simulink model "OnlineEstimation_MIL"  (R2024a)
settings: Solver=FixedStepAuto  StartTime=0.0  StopTime=50  FixedStep=0.001  RelTol=1e-3
undefined symbols (not defined in the file or in its folder): magnitude
libraries: fl_lib x16, nesl_utility x10, simulink x4, ee_lib x4, fl_ps_legacy_lib x2, ctrlSharedLib x2, eeGeneralControl x2, sdl_lib x1
settings Model: Creator=rocke  LastModifiedBy=rocke

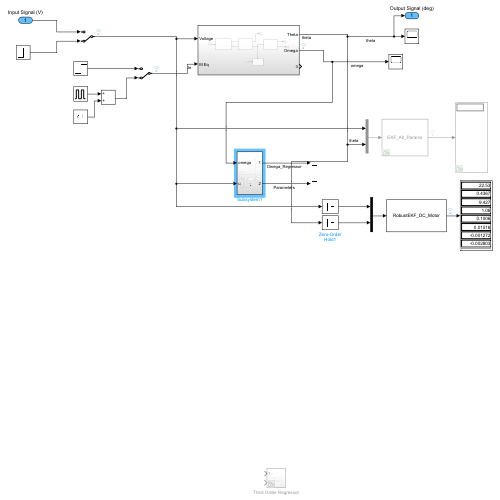
[thumbnail: Simulink's stored preview of the top-level diagram]
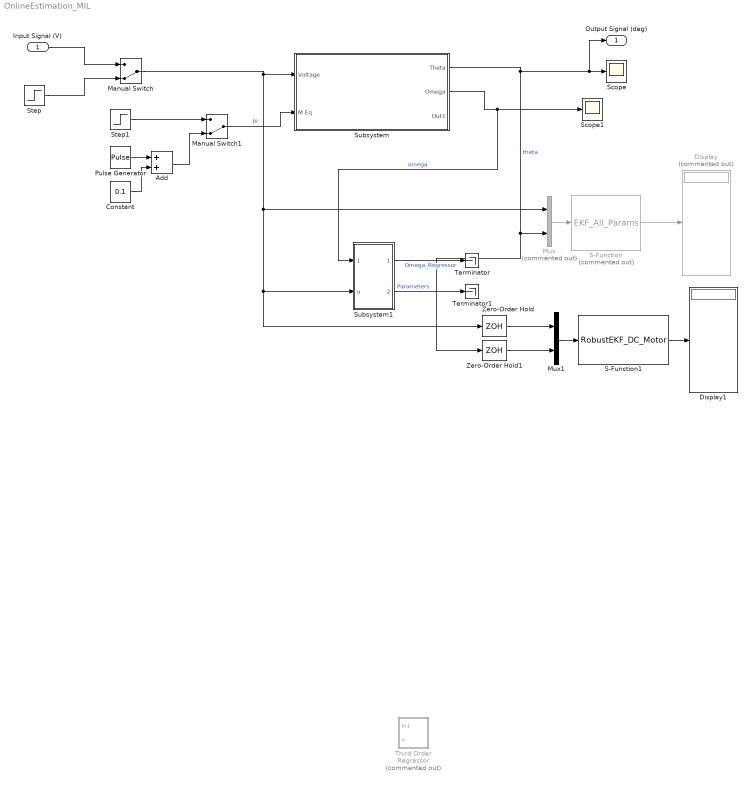
== system OnlineEstimation_MIL ==
  Input Signal (V) : Inport
  Add : Sum
  Constant : Constant  Value=0.1
  Display : Display  Commented=on
  Display1 : Display
  Manual Switch : ManualSwitch  CurrentSetting=0
  Manual Switch1 : ManualSwitch  CurrentSetting=0
  Mux : Mux  Commented=on  Inputs=2
  Mux1 : Mux  Inputs=2
  Pulse Generator : DiscretePulseGenerator  PulseType=Time based  Amplitude=0.2  Period=10  PulseWidth=50  PhaseDelay=5
  S-Function : S-Function  Commented=on  FunctionName=EKF_All_Params  SFunctionDeploymentMode=off  EnableBusSupport=off
  S-Function1 : S-Function  FunctionName=RobustEKF_DC_Motor  SFunctionDeploymentMode=off  EnableBusSupport=off
  Scope : Scope
  Scope1 : Scope
  Step : Step  Time=2  After=12  SampleTime=0
  Step1 : Step  Time=5  Before=0.1  After=0.2  SampleTime=0
  Subsystem : Subsystem
  Subsystem1 : Subsystem
  Terminator : Terminator
  Terminator1 : Terminator
  Third Order Regressor : Subsystem  Commented=on
  Zero-Order Hold : ZeroOrderHold  SampleTime=-1
  Zero-Order Hold1 : ZeroOrderHold  SampleTime=-1
  Output Signal (deg) : Outport  VectorParamsAs1DForOutWhenUnconnected=off
  wires:
  Input Signal (V)/1 -> Manual Switch/1
  Step/1 -> Manual Switch/2
  Manual Switch1/1 -> Subsystem/2(M Eq)  "Je"
  Subsystem/2(Omega) -> Subsystem1/1(omega), Scope1/1  "omega"
  Mux/1 -> S-Function/1
  S-Function/1 -> Display/1
  Manual Switch/1 -> Zero-Order Hold/1, Subsystem1/2(u), Mux/1, Subsystem/1(Voltage)
  Subsystem/1(Theta) -> Mux/2, Zero-Order Hold1/1, Scope/1, Output Signal (deg)/1  "theta"
  S-Function1/1 -> Display1/1
  Mux1/1 -> S-Function1/1
  Zero-Order Hold/1 -> Mux1/1
  Zero-Order Hold1/1 -> Mux1/2
  Step1/1 -> Manual Switch1/1
  Pulse Generator/1 -> Add/1
  Add/1 -> Manual Switch1/2
  Constant/1 -> Add/2
  Subsystem1/1(Out1) -> Terminator/1  "Omega_Regressor"
  Subsystem1/2(Out2) -> Terminator1/1  "Parameters"

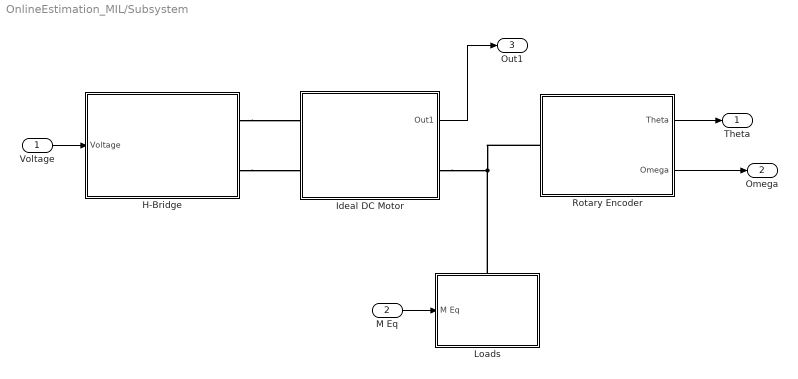
== system OnlineEstimation_MIL/Subsystem ==
  Voltage : Inport
  M Eq : Inport  Port=2
  H-Bridge : Subsystem
      mask Display: image('H-Bridge.jpg', [5,0,1,0,100,100]);
  Ideal DC Motor : Subsystem
      mask Display: image('DC_Motor.jpg', [1,0,1,0,100,100]);
  Loads : Subsystem
      settings: PortSchema="{\"entries\":[{\"content\":{\"sides\":[{\"content\":{\"connectorIds\":[\"In1\"]},\"type\":\"ConnectorPlacement.EquallySpacedRectSide\",\"uuid\":\"35af7967-d601-467b-871c-2decdb5f576d\"},{\"content\":{\"side\":\"RIGHT\"},\"type\":\"ConnectorPlacement.EquallySpacedRectSide\",\"uuid\":\"f82d529b-61c3-41a9-ad40-44f1ee2700d7\"},{\"content\":{\"connectorIds\":[\"LConn1\"],\"side\":\"TOP\"},\"type\":\"ConnectorPlacement.EquallySpacedRectSide\",\"uuid\":\"077b85ac-e334-479f-9bfe-5c63e4ba6a3d\"}]},\"type\":\"ConnectorPlacement.EquallySpacedConnector\",\"uuid\":\"d8fe6e45-beb6-425e-8bfa-63ec555f59a4\"}],\"packageUris\":[\"http://schema.mathworks.com/mf0/Connector/R2020b\"],\"version\":\"1.0\"}"
  Rotary Encoder : Subsystem
      mask Display: image('Rotary_Encoder.jpg', [1,0,1,0,100,100]);
  Theta : Outport
  Omega : Outport  Port=2
  Out1 : Outport  Port=3
  wires:
  Rotary Encoder/2(Omega) -> Omega/1
  M Eq/1 -> Loads/1(M Eq)
  Rotary Encoder/1(Theta) -> Theta/1
  Voltage/1 -> H-Bridge/1(Voltage)
  Ideal DC Motor/1(Out1) -> Out1/1
  connections:
  Ideal DC Motor/RConn1 -- Rotary Encoder/LConn1 -- Loads/LConn1
  H-Bridge/RConn1 -- Ideal DC Motor/LConn1
  H-Bridge/RConn2 -- Ideal DC Motor/LConn2

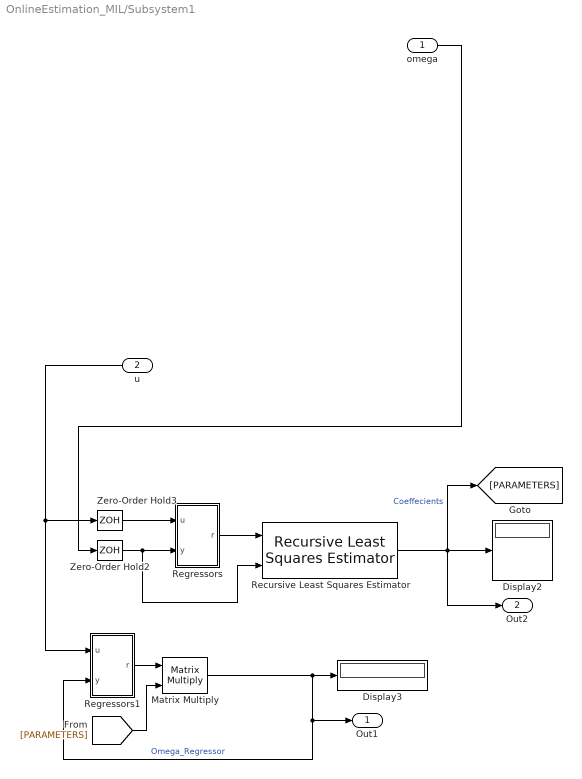
== system OnlineEstimation_MIL/Subsystem1 ==
  omega : Inport
  u : Inport  Port=2
  Display2 : Display
  Display3 : Display
  Matrix Multiply : Product  Multiplication=Matrix(*)
  Recursive Least Squares Estimator : ctrlSharedLib/Recursive Least Squares Estimator  InitialEstimateSource=Internal  InitialParameterData=[0 0.4 -0.25]  P0=1e4  InitialRegressors=0  InitialOutputs=0  History=Infinite  WindowLength=200  EstimationMethod=Forgetting Factor  AdaptationParameter=0.98  HasTimeVaryingAdaptationParameter=off  NormalizationBias=eps  OutputError=off  OutputP=off  AddEnablePort=off  InputProcessing=Sample-based  Ts=-1
      settings: LibrarySourceBlock=slident/Estimators/Recursive Least Squares Estimator
  Regressors : Subsystem
  Regressors1 : Subsystem
  Zero-Order Hold2 : ZeroOrderHold  SampleTime=0.001
  Zero-Order Hold3 : ZeroOrderHold  SampleTime=0.001
  Out1 : Outport
  Out2 : Outport  Port=2
  wires:
  Zero-Order Hold3/1 -> Regressors/1(u)
  Matrix Multiply/1 -> Display3/1, Out1/1, Regressors1/2(y)  "Omega_Regressor"
  Regressors/1(r) -> Recursive Least Squares Estimator/1
  Recursive Least Squares Estimator/1 -> Out2/1, [PARAMETERS], Display2/1  "Coeffecients"
  u/1 -> Regressors1/1(u), Zero-Order Hold3/1
  Regressors1/1(r) -> Matrix Multiply/1
  Zero-Order Hold2/1 -> Regressors/2(y), Recursive Least Squares Estimator/2
  [PARAMETERS] -> Matrix Multiply/2
  omega/1 -> Zero-Order Hold2/1

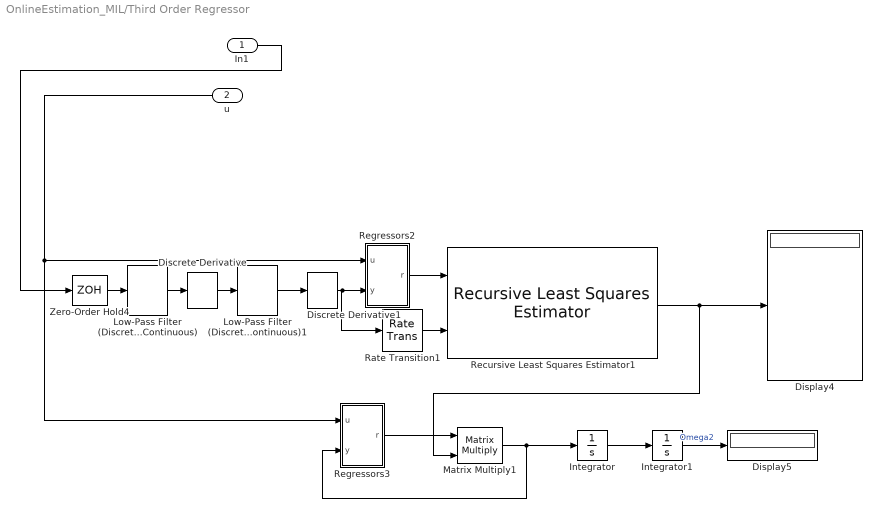
== system OnlineEstimation_MIL/Third Order Regressor ==
  In1 : Inport
  u : Inport  Port=2
  Discrete Derivative : simulink/Discrete/Discrete Derivative  gainval=1.0  ICPrevScaledInput=0.0  OutMin=[]  OutMax=[]  OutDataType=fixdt(1, 16)  OutScaling=2^-10  DoSatur=off
  Discrete Derivative1 : simulink/Discrete/Discrete Derivative  gainval=1.0  ICPrevScaledInput=0.0  OutMin=[]  OutMax=[]  OutDataType=fixdt(1, 16)  OutScaling=2^-10  DoSatur=off
  Display4 : Display
  Display5 : Display
  Integrator : Integrator
  Integrator1 : Integrator
  Low-Pass Filter (Discrete or Continuous) : eeGeneralControl/Low-Pass Filter (Discrete or Continuous)  K=1  T=0.1  B=inf  A=-inf  init_option=Inherited from block input  x0=0  Ts=-1
  Low-Pass Filter (Discrete or Continuous)1 : eeGeneralControl/Low-Pass Filter (Discrete or Continuous)  K=1  T=0.1  B=inf  A=-inf  init_option=Inherited from block input  x0=0  Ts=-1
  Matrix Multiply1 : Product  Multiplication=Matrix(*)
  Rate Transition1 : RateTransition  OutPortSampleTime=0.001
  Recursive Least Squares Estimator1 : ctrlSharedLib/Recursive Least Squares Estimator  InitialEstimateSource=None  InitialParameterData=3  P0=1e4  InitialRegressors=0  InitialOutputs=0  History=Infinite  WindowLength=200  EstimationMethod=Kalman Filter  AdaptationParameter=1  HasTimeVaryingAdaptationParameter=off  NormalizationBias=eps  OutputError=off  OutputP=off  AddEnablePort=off  InputProcessing=Sample-based  Ts=-1
      settings: LibrarySourceBlock=slident/Estimators/Recursive Least Squares Estimator
  Regressors2 : Subsystem
  Regressors3 : Subsystem
  Zero-Order Hold4 : ZeroOrderHold  SampleTime=0.001
  wires:
  Regressors2/1(r) -> Recursive Least Squares Estimator1/1
  Regressors3/1(r) -> Matrix Multiply1/1
  Matrix Multiply1/1 -> Regressors3/2(y), Integrator/1
  Recursive Least Squares Estimator1/1 -> Matrix Multiply1/2, Display4/1
  Rate Transition1/1 -> Recursive Least Squares Estimator1/2
  Integrator1/1 -> Display5/1  "Omega2"
  u/1 -> Regressors2/1(u), Regressors3/1(u)
  Discrete Derivative1/1 -> Rate Transition1/1, Regressors2/2(y)
  Integrator/1 -> Integrator1/1
  Discrete Derivative/1 -> Low-Pass Filter (Discrete or Continuous)1/1
  Low-Pass Filter (Discrete or Continuous)/1 -> Discrete Derivative/1
  Low-Pass Filter (Discrete or Continuous)1/1 -> Discrete Derivative1/1
  Zero-Order Hold4/1 -> Low-Pass Filter (Discrete or Continuous)/1
  In1/1 -> Zero-Order Hold4/1

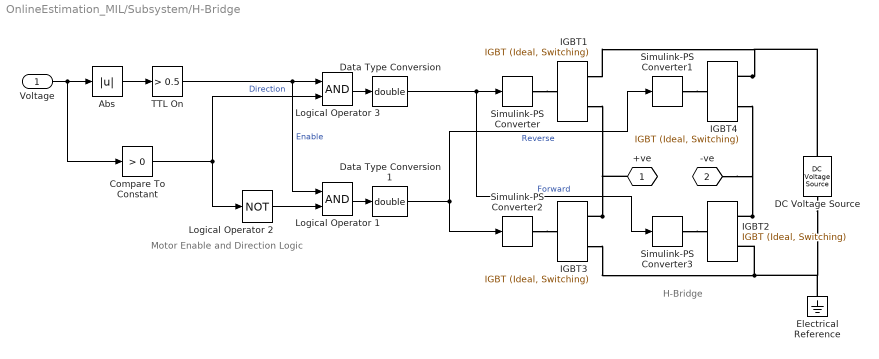
== system OnlineEstimation_MIL/Subsystem/H-Bridge ==
  note: Motor Enable and Direction Logic
  note: H-Bridge
  Voltage : Inport
  Abs : Abs  SaturateOnIntegerOverflow=off
  Compare To Constant : simulink/Logic and Bit Operations/Compare To Constant  relop=>  const=0  OutDataTypeStr=boolean  ZeroCross=off
  DC Voltage Source : fl_lib/Electrical/Electrical Sources/DC Voltage Source  v0=12 V
  Data Type Conversion : DataTypeConversion  OutDataTypeStr=double  SaturateOnIntegerOverflow=off  RndMeth=Floor
  Data Type Conversion1 : DataTypeConversion  OutDataTypeStr=double  SaturateOnIntegerOverflow=off  RndMeth=Floor
  Electrical Reference : fl_lib/Electrical/Electrical Elements/Electrical Reference
  IGBT{1..4} (4 alike) : ee_lib/Semiconductors & Converters/IGBT (Ideal, Switching)  port_option=ee.enum.controlport.ps  Vf=1 V  Ron=0.001 Ohm  Goff=1e-5 1/Ohm  Vth=0.5 V  diode_param=1  diode_Vf=0.8 V  diode_Ron=0.001 Ohm  diode_Goff=1e-5 1/Ohm  diode_C=5e-8 F  diode_iRM=-235 A  diode_iF=300 A  diode_idot=-50 A/us  diode_trr_param=1  diode_trr_factor=3  diode_trr=15 us  diode_Qrr=1.5e+3 s*uA  ice_specify=off  ice_priority=None  ice=0 A  ice_nominal_specify=off  ice_nominal_value=1  ice_nominal_unit=A  vce_specify=off  vce_priority=None  vce=0 V  vce_nominal_specify=off  vce_nominal_value=1  vce_nominal_unit=V  vge_specify=off  vge_priority=None  vge=0 V  vge_nominal_specify=off  vge_nominal_value=1  vge_nominal_unit=V  thermal_loss_option=ee.enum.converters.thermalLossOption.constantvalues  Von_data=[0, .1, .6, .8, 1, 1.3, 1.6, 2, 2.4; 0, .1, .7, 1, 1.2, 1.5, 1.9, 2.4, 2.8] V  Tj=[298.15, 398.15] K  Iout_data=[0, .1, 1, 5, 10, 20, 40, 70, 100] A  Eon_data=[0, .0024, .024, .12, .2, .48, 1.04, 2.16, 3.24; 0, .003, .03, .15, .25, .6, 1.3, 2.7, 4.05] * 1e-3 J  Eoff_data=[0, .0007, .0066, .033, .066, .17, .33, .83, 1.5; 0, .001, .01, .05, .1, .25, .5, 1.2, 2.2] * 1e-3 J  Eon_data_3D=[zeros(2, 9, 3)] J  Eoff_data_3D=[zeros(2, 9, 3)] J  Tj_loss=[298.15, 398.15] K  Iout_data_loss=[0, .1, 1, 5, 10, 20, 40, 70, 100] A  tabulateWithVce=false  Vce_loss=[0, 150, 300] V  Eon_scalar=22.86e-3 J  Eoff_scalar=17.14e-3 J  Voff=300 V  Iout_scalar=600 A  useCurrentFromPreviousCycle=false  useVoltageFromPreviousCycle=false  diodeModelType=ee.enum.converters.diodeModelType.pwl  diodeTableType=ee.enum.diode.tableType.IfMat  diode_ReverseIVType=ee.enum.diode.diodeReverseIV.constant  diode_IfMat=[.07, .12, .19, 1.75, 4.24, 7.32, 11.2; .16, .3, .72, 2.14, 4.02, 6.35, 9.12] A  diode_VfMat=[.9, 1.15, 1.25, 1.5, 1.75, 2.17, 2.6, 2.85; .58, .68, .75, 1.1, 1.38, 1.77, 2.27, 2.7] V  diode_TjVec=[25, 125] degC  diode_VfVec=[.5, .7, .9, 1.3, 1.7, 2.1, 2.5] V  diode_IfVec=[.1, .2, .5, 1, 2, 4, 7, 10] A  diode_IrMat=[1e-06, 2e-06, 5e-06, 1e-05, 2.5e-05, 5e-05, .0001; 2e-06, 5e-06, 1e-05, 4e-05, 8e-05, .0002, .0005] A  diode_VrMat=[10, 100, 200, 250, 300, 325, 350; 10, 70, 160, 220, 270, 300, 320] V  diode_VrVec=[10, 20, 40, 50, 70, 80, 100] V  diode_IrVec=[1e-06, 2e-06, 5e-06, 1e-05, 2e-05, 5e-05, .0001] A  diode_Vr=-600 V  diode_Ls=150 nH  diode_Erec=0.03 J  diode_rec_loss_model=ee.enum.diode.reverseRecoveryModel.fixed  diode_ErecVal=0 J  diode_scaleWithIandV=true  diode_ErecMat=zeros(2, 3) J  diode_TjrecVec=[298.15, 398.15] K  diode_IfrecVec=[.1, 1, 10] A  diode_IrecVal=10 A  diode_VrecVal=10 V  diode_tFilter=1 / 1000 / 100 s  thermal_network_parameterization=ee.enum.thermalNetworkTopology.external  Rth=[.08, .5] K/W  Rth_Cauer=[.08, .1, .5] K/W  Rth_Foster=[.08, .14, .22, .16] K/W  thermal_mass_parameterization=ee.enum.thermalNetwork.timeconstant  thermal_mass=[.01, .5] J/K  thermal_mass_Cauer=[.01, .1, .5] J/K  thermal_mass_Foster=[.001, .005, .05, .5] J/K  thermal_time_constant=[.001, .2] s  thermal_time_constant_Cauer=[.001, .1, .2] s  thermal_time_constant_Foster=[7e-05, .0007, .01, .08] s  thermal_mass_initial_temperatures=[25, 25] degC  thermal_mass_initial_temperatures_Cauer=[25, 25, 25] degC  junction_thermal_mass=0.01 J/K  Tvec_initial_Foster=[25, 25, 25, 25] degC  no_thermal_network=0  junction_temperature_specify=off  junction_temperature_priority=None  junction_temperature=25 degC  junction_temperature_nominal_specify=off  junction_temperature_nominal_value=1  junction_temperature_nominal_unit=degC  Qj_specify=off  Qj_priority=None  Qj=0 W  Qj_nominal_specify=off  Qj_nominal_value=1  Qj_nominal_unit=W  accumulatedSwitchingLosses_specify=off  accumulatedSwitchingLosses_priority=None  accumulatedSwitchingLosses=0 J
  Logical Operator 1 : Logic  AllPortsSameDT=off  OutDataTypeStr=boolean
  Logical Operator 2 : Logic  Operator=NOT  AllPortsSameDT=off  OutDataTypeStr=boolean
  Logical Operator 3 : Logic  AllPortsSameDT=off  OutDataTypeStr=boolean
  Simulink-PS Converter{,1..3} (4 alike) : nesl_utility/Simulink-PS Converter  PhysicalDomain=network_engine_domain  SubClassName=ps_input  LeftPortType=input  RightPortType=output  PseudoPeriodic=off  Frequencies=[]  NoiseDistribution=none  NoiseParameters=[]  Unit=1  AffineConversion=off  FilteringAndDerivatives=provide  SimscapeFilterOrder=1  InputFilterTimeConstant=0.001  UdotUserProvided=0
  TTL On : simulink/Logic and Bit Operations/Compare To Constant  relop=>  const=0.5  OutDataTypeStr=boolean  ZeroCross=off
  +ve : PMIOPort  Tag=PMCPort  Side=Right
  -ve : PMIOPort  Tag=PMCPort  Port=2  Side=Right
  wires:
  Data Type Conversion1/1 -> Simulink-PS Converter1/1, Simulink-PS Converter2/1  "Reverse"
  Data Type Conversion/1 -> Simulink-PS Converter3/1, Simulink-PS Converter/1  "Forward"
  Abs/1 -> TTL On/1
  TTL On/1 -> Logical Operator 3/1, Logical Operator 1/1  "Enable"
  Voltage/1 -> Abs/1, Compare To Constant/1
  Compare To Constant/1 -> Logical Operator 3/2, Logical Operator 2/1  "Direction"
  Logical Operator 2/1 -> Logical Operator 1/2
  Logical Operator 3/1 -> Data Type Conversion/1
  Logical Operator 1/1 -> Data Type Conversion1/1
  connections:
  Simulink-PS Converter/RConn1 -- IGBT1/LConn1
  Simulink-PS Converter1/RConn1 -- IGBT4/LConn1
  Simulink-PS Converter2/RConn1 -- IGBT3/LConn1
  Simulink-PS Converter3/RConn1 -- IGBT2/LConn1
  IGBT4/RConn1 -- IGBT1/RConn1 -- DC Voltage Source/LConn1
  IGBT3/RConn1 -- IGBT1/RConn2 -- +ve/RConn1
  IGBT3/RConn2 -- IGBT2/RConn2 -- DC Voltage Source/RConn1 -- Electrical Reference/LConn1
  IGBT2/RConn1 -- IGBT4/RConn2 -- -ve/RConn1

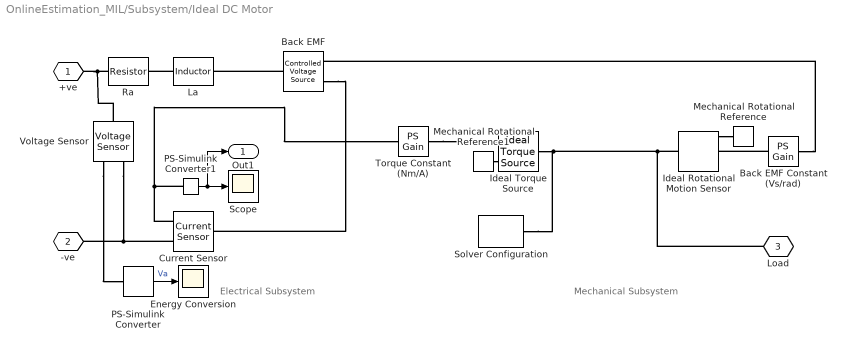
== system OnlineEstimation_MIL/Subsystem/Ideal DC Motor ==
  note: Electrical
      | Subsystem
  note: Mechanical
      | Subsystem
  Back EMF : fl_lib/Electrical/Electrical Sources/Controlled Voltage Source
  Back EMF Constant (Vs/rad) : fl_ps_legacy_lib/Legacy Physical Signals/Functions/PS Gain  gain=0.01
  Current Sensor : fl_lib/Electrical/Electrical Sensors/Current Sensor
  Energy Conversion : Scope
  Ideal Rotational Motion Sensor : fl_lib/Mechanical/Mechanical Sensors/Ideal Rotational Motion Sensor  reference=foundation.enum.MeasurementReference.difference  acceleration_port=false  velocity_port=true  position_port=true  wrap_angle=simscape.enum.onoff.off  offset=0 rad
  Ideal Torque Source : fl_lib/Mechanical/Mechanical Sources/Ideal Torque Source
  La : fl_lib/Electrical/Electrical Elements/Inductor  l=0.5 H  r=0 Ohm  g=0 1/Ohm  i_specify=off  i_priority=None  i=0 A  i_nominal_specify=off  i_nominal_value=1  i_nominal_unit=A  v_specify=off  v_priority=None  v=0 V  v_nominal_specify=off  v_nominal_value=1  v_nominal_unit=V  i_L_specify=off  i_L_priority=High  i_L=0 A  i_L_nominal_specify=off  i_L_nominal_value=1  i_L_nominal_unit=A
  Mechanical Rotational Reference : fl_lib/Mechanical/Rotational Elements/Mechanical Rotational Reference
  Mechanical Rotational Reference1 : fl_lib/Mechanical/Rotational Elements/Mechanical Rotational Reference
  PS-Simulink Converter : nesl_utility/PS-Simulink Converter  PhysicalDomain=network_engine_domain  SubClassName=ps_output  LeftPortType=input  RightPortType=output  PseudoPeriodic=off  Frequencies=[]  VectorFormat=1-D array  Unit=1  AffineConversion=off
  PS-Simulink Converter1 : nesl_utility/PS-Simulink Converter  PhysicalDomain=network_engine_domain  SubClassName=ps_output  LeftPortType=input  RightPortType=output  PseudoPeriodic=off  Frequencies=[]  VectorFormat=inherit  Unit=inherit  AffineConversion=off
  Ra : fl_lib/Electrical/Electrical Elements/Resistor  R=2 Ohm  i_specify=off  i_priority=None  i=0 A  i_nominal_specify=off  i_nominal_value=1  i_nominal_unit=A  v_specify=off  v_priority=None  v=0 V  v_nominal_specify=off  v_nominal_value=1  v_nominal_unit=V
  Scope : Scope
  Solver Configuration : nesl_utility/Solver Configuration  PhysicalDomain=network_engine_domain  SubClassName=solver  LeftPortType=input  RightPortType=generic  Tones=[]  Harmonics=[]  SimulateNoise=off  Profile=off  UseLocalSampling=off  EnableSwitchedLinearOptims=on  FrequencyDomain=off  UseCCode=off  RelTol=0.001  AbsTol=1e-06  MinStep=1e-09  ToWorkspace=off  RevertToSquareIcSolve=off  NumHomotopyIterations=100  PhasorMode=off  PhasorModeNumHarmonics=1  ConsistencySolver=NEWTON_FTOL  IndexReductionMethod=DerivativeReplacement  DoDC=off  ResidualTolerance=1e-9  ConsistencyTolSource=GLOBAL  ConsistencyAbsTol=0.001  ConsistencyRelTol=0.001  ConsistencyTolFactor=0.001  UseLocalSolver=off  LocalSolverChoice=NE_BACKWARD_EULER_ADVANCER  ResolveIndetEquations=on  FunctionEvalNumThread=1  LocalSolverSampleTime=.001  DoFixedCost=off  MaxNonlinIter=3  MaxModeIter=2  ComputeImpulses=off  ImpulseIterations=2  LinearAlgebra=Sparse  LinearAlgebraNumThread=0  EquationFormulation=NE_TIME_EF  DelaysMemoryBudget=1024  AutomaticFiltering=on  FilteringTimeConstant=0.001  PartitionStorageMethod=AS_NEEDED  PartitionMemoryBudget=1024  PartitionMethod=FAST  MultibodyUseLocalSolver=off  MultibodyLocalSolverChoice=ODE1  MultibodyLocalSolverSampleTime=0.001
  Torque Constant (Nm/A) : fl_ps_legacy_lib/Legacy Physical Signals/Functions/PS Gain  gain=0.01
  Voltage Sensor : fl_lib/Electrical/Electrical Sensors/Voltage Sensor
  +ve : PMIOPort  Tag=PMCPort  Side=Left
  -ve : PMIOPort  Tag=PMCPort  Port=2  Side=Left
  Load : PMIOPort  Port=3  Side=Right
  Out1 : Outport
  wires:
  PS-Simulink Converter/1 -> Energy Conversion/1  "Va"
  PS-Simulink Converter1/1 -> Out1/1, Scope/1
  connections:
  La/LConn1 -- Ra/RConn1
  Ideal Rotational Motion Sensor/LConn1 -- Ideal Torque Source/LConn1 -- Solver Configuration/RConn1 -- Load/RConn1
  Back EMF Constant (Vs/rad)/LConn1 -- Ideal Rotational Motion Sensor/RConn2
  Ideal Rotational Motion Sensor/RConn1 -- Mechanical Rotational Reference/LConn1
  Mechanical Rotational Reference1/LConn1 -- Ideal Torque Source/RConn2
  Torque Constant (Nm/A)/RConn1 -- Ideal Torque Source/RConn1
  Back EMF/LConn1 -- La/RConn1
  Back EMF/RConn2 -- Current Sensor/LConn1
  Current Sensor/RConn2 -- Voltage Sensor/RConn2 -- -ve/RConn1
  Current Sensor/RConn1 -- PS-Simulink Converter1/LConn1 -- Torque Constant (Nm/A)/LConn1
  Back EMF Constant (Vs/rad)/RConn1 -- Back EMF/RConn1
  Voltage Sensor/RConn1 -- PS-Simulink Converter/LConn1
  Ra/LConn1 -- Voltage Sensor/LConn1 -- +ve/RConn1

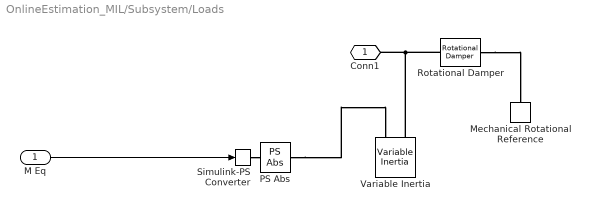
== system OnlineEstimation_MIL/Subsystem/Loads ==
  M Eq : Inport
  Mechanical Rotational Reference : fl_lib/Mechanical/Rotational Elements/Mechanical Rotational Reference
  PS Abs : fl_lib/Physical Signals/Nonlinear Operators/PS Abs
      settings: InternalSimscapePortConfiguration="{\"Bottom\":[],\"Left\":[{\"id\":\"I\",\"label\":\"\",\"type\":\"input\"}],\"Right\":[{\"id\":\"O\",\"label\":\"\",\"type\":\"output\"}],\"Top\":[]}"
  Rotational Damper : fl_lib/Mechanical/Rotational Elements/Rotational Damper  D=0.1 N*m*s/rad  w_specify=off  w_priority=None  w=0 rad/s  w_nominal_specify=off  w_nominal_value=1  w_nominal_unit=rad/s  t_specify=off  t_priority=None  t=0 N*m  t_nominal_specify=off  t_nominal_value=1  t_nominal_unit=N*m
  Simulink-PS Converter : nesl_utility/Simulink-PS Converter  PhysicalDomain=network_engine_domain  SubClassName=ps_input  LeftPortType=input  RightPortType=output  PseudoPeriodic=off  Frequencies=[]  NoiseDistribution=none  NoiseParameters=[]  Unit=1  AffineConversion=off  FilteringAndDerivatives=filter  SimscapeFilterOrder=1  InputFilterTimeConstant=0.001  UdotUserProvided=0
  Variable Inertia : sdl_lib/Inertias & Loads/Variable Inertia  minimum_inertia=0.0001 kg*m^2  L_specify=off  L_priority=High  L=0 kg*m^2/s  L_nominal_specify=off  L_nominal_value=1  L_nominal_unit=kg*m^2/s
      settings: InternalSimscapePortConfiguration="{\"Bottom\":[],\"Left\":[{\"id\":\"I\",\"label\":\"\",\"type\":\"input\"},{\"id\":\"A\",\"label\":\"\",\"type\":\"foundation.mechanical.rotational.rotational\"}],\"Right\":[],\"Top\":[]}"
  Conn1 : PMIOPort  Side=Left
  wires:
  M Eq/1 -> Simulink-PS Converter/1
  connections:
  Simulink-PS Converter/RConn1 -- PS Abs/LConn1
  PS Abs/RConn1 -- Variable Inertia/LConn1
  Variable Inertia/LConn2 -- Rotational Damper/LConn1 -- Conn1/RConn1
  Rotational Damper/RConn1 -- Mechanical Rotational Reference/LConn1

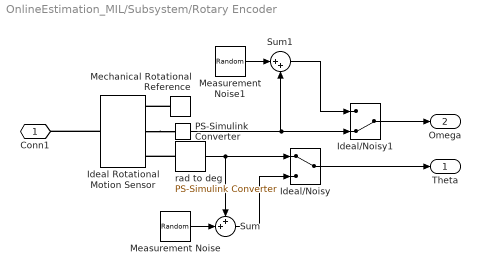
== system OnlineEstimation_MIL/Subsystem/Rotary Encoder ==
  Ideal Rotational Motion Sensor : fl_lib/Mechanical/Mechanical Sensors/Ideal Rotational Motion Sensor  reference=foundation.enum.MeasurementReference.difference  acceleration_port=false  velocity_port=true  position_port=true  wrap_angle=false  offset=0 rad
  Ideal/Noisy : ManualSwitch
  Ideal/Noisy1 : ManualSwitch  CurrentSetting=0
  Measurement Noise : RandomNumber  Variance=0.001  SampleTime=0.01
  Measurement Noise1 : RandomNumber  Variance=0.0001  SampleTime=0.01
  Mechanical Rotational Reference : fl_lib/Mechanical/Rotational Elements/Mechanical Rotational Reference
  PS-Simulink Converter : nesl_utility/PS-Simulink Converter  PhysicalDomain=network_engine_domain  SubClassName=ps_output  LeftPortType=input  RightPortType=output  PseudoPeriodic=off  Frequencies=[]  VectorFormat=inherit  Unit=inherit  AffineConversion=off
  Sum : Sum  Inputs=++|
  Sum1 : Sum  Inputs=|++
  rad to deg : nesl_utility/PS-Simulink Converter  PhysicalDomain=network_engine_domain  SubClassName=ps_output  LeftPortType=input  RightPortType=output  PseudoPeriodic=off  Frequencies=[]  VectorFormat=1-D array  Unit=rad  AffineConversion=off
  Conn1 : PMIOPort  Side=Left
  Theta : Outport
  Omega : Outport  Port=2
  wires:
  rad to deg/1 -> Sum/1, Ideal/Noisy/1
  Measurement Noise/1 -> Sum/2
  Sum/1 -> Ideal/Noisy/2
  Ideal/Noisy/1 -> Theta/1
  Ideal/Noisy1/1 -> Omega/1
  Sum1/1 -> Ideal/Noisy1/1
  Measurement Noise1/1 -> Sum1/1
  PS-Simulink Converter/1 -> Sum1/2, Ideal/Noisy1/2
  connections:
  Mechanical Rotational Reference/LConn1 -- Ideal Rotational Motion Sensor/RConn1
  rad to deg/LConn1 -- Ideal Rotational Motion Sensor/RConn3
  Ideal Rotational Motion Sensor/LConn1 -- Conn1/RConn1
  Ideal Rotational Motion Sensor/RConn2 -- PS-Simulink Converter/LConn1

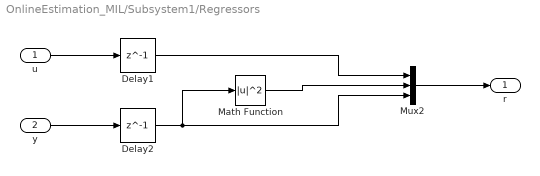
== system OnlineEstimation_MIL/Subsystem1/Regressors ==
  u : Inport
  y : Inport  Port=2
  Delay1 : Delay  DelayLength=1  InitialCondition=1  SampleTime=0.001
  Delay2 : Delay  DelayLength=1  InitialCondition=2  SampleTime=0.001
  Math Function : Math  Operator=magnitude^2  SignedPower=on
  Mux2 : Mux  Inputs=3
  r : Outport  VectorParamsAs1DForOutWhenUnconnected=off
  wires:
  u/1 -> Delay1/1
  Mux2/1 -> r/1
  y/1 -> Delay2/1
  Delay1/1 -> Mux2/1
  Math Function/1 -> Mux2/2
  Delay2/1 -> Math Function/1, Mux2/3

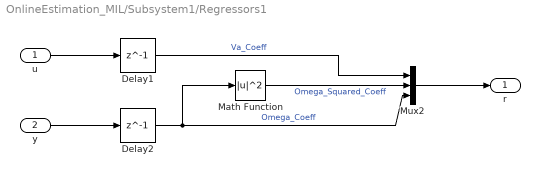
== system OnlineEstimation_MIL/Subsystem1/Regressors1 ==
  u : Inport
  y : Inport  Port=2
  Delay1 : Delay  DelayLength=1  InitialCondition=1  SampleTime=0.001
  Delay2 : Delay  DelayLength=1  InitialCondition=2  SampleTime=0.001
  Math Function : Math  Operator=magnitude^2  SignedPower=on
  Mux2 : Mux  Inputs=3
  r : Outport  VectorParamsAs1DForOutWhenUnconnected=off
  wires:
  u/1 -> Delay1/1
  Mux2/1 -> r/1
  y/1 -> Delay2/1
  Delay1/1 -> Mux2/1  "Va_Coeff"
  Math Function/1 -> Mux2/2  "Omega_Squared_Coeff"
  Delay2/1 -> Math Function/1, Mux2/3  "Omega_Coeff"

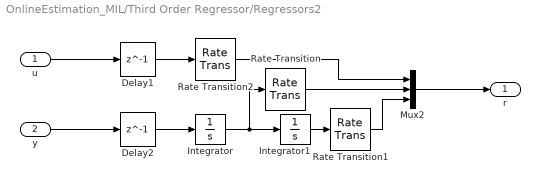
== system OnlineEstimation_MIL/Third Order Regressor/Regressors2 ==
  u : Inport
  y : Inport  Port=2
  Delay1 : Delay  DelayLength=1  InitialCondition=1  SampleTime=0.001
  Delay2 : Delay  DelayLength=1  InitialCondition=2  SampleTime=0.001
  Integrator : Integrator
  Integrator1 : Integrator
  Mux2 : Mux  Inputs=3
  Rate Transition : RateTransition  OutPortSampleTime=0.001
  Rate Transition1 : RateTransition  OutPortSampleTime=0.001
  Rate Transition2 : RateTransition  OutPortSampleTime=0.001
  r : Outport  VectorParamsAs1DForOutWhenUnconnected=off
  wires:
  u/1 -> Delay1/1
  Mux2/1 -> r/1
  y/1 -> Delay2/1
  Delay1/1 -> Rate Transition2/1
  Integrator/1 -> Integrator1/1, Rate Transition/1
  Delay2/1 -> Integrator/1
  Integrator1/1 -> Rate Transition1/1
  Rate Transition/1 -> Mux2/2
  Rate Transition1/1 -> Mux2/3
  Rate Transition2/1 -> Mux2/1

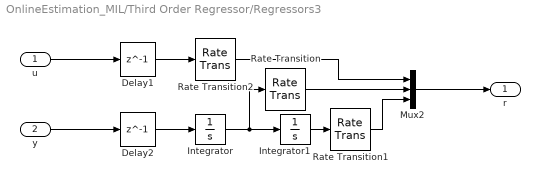
== system OnlineEstimation_MIL/Third Order Regressor/Regressors3 ==
  u : Inport
  y : Inport  Port=2
  Delay1 : Delay  DelayLength=1  InitialCondition=1  SampleTime=0.001
  Delay2 : Delay  DelayLength=1  InitialCondition=2  SampleTime=0.001
  Integrator : Integrator
  Integrator1 : Integrator
  Mux2 : Mux  Inputs=3
  Rate Transition : RateTransition  OutPortSampleTime=0.001
  Rate Transition1 : RateTransition  OutPortSampleTime=0.001
  Rate Transition2 : RateTransition  OutPortSampleTime=0.001
  r : Outport  VectorParamsAs1DForOutWhenUnconnected=off
  wires:
  u/1 -> Delay1/1
  Mux2/1 -> r/1
  y/1 -> Delay2/1
  Delay1/1 -> Rate Transition2/1
  Integrator/1 -> Integrator1/1, Rate Transition/1
  Delay2/1 -> Integrator/1
  Integrator1/1 -> Rate Transition1/1
  Rate Transition/1 -> Mux2/2
  Rate Transition1/1 -> Mux2/3
  Rate Transition2/1 -> Mux2/1
